simulink model "counter"  (R2021a)
settings: Solver=FixedStepDiscrete  StartTime=0.0  StopTime=10.0  RelTol=1e-3  EnableMultiTasking=on
settings Model: Creator=Noha  LastModifiedBy=Noha
settings DataIOCC: ReturnWorkspaceOutputs=off
settings OptimizationCC: DefaultParameterBehavior=Inlined  InlineInvariantSignals=on  EnableMemcpy=off  LifeSpan=1  EfficientTunableParamExpr=on
settings DebuggingCC: UnderspecifiedInitializationDetection=Classic  MergeDetectMultiDrivingBlocksExec=none  SFMachineParentedDataDiag=warning  ArithmeticOperatorsInVariantConditions=warning
settings ModelReferenceCC: PropagateSignalLabelsOutOfModel=off
settings SFSimCC: MATLABDynamicMemAlloc=off  CustomCodeUndefinedFunction=UseInterfaceOnly
settings RTWCC: SystemTargetFile=ert.tlc  GenCodeOnly=on  TemplateMakefile=ert_default_tmf  GenerateReport=on  IncludeHyperlinkInReport=on  LaunchReport=on  GenerateTraceInfo=on  GenerateTraceReport=on  GenerateTraceReportSl=on  GenerateTraceReportSf=on  GenerateTraceReportEml=on
settings CodeAppCC: ForceParamTrailComments=on  IgnoreCustomStorageClasses=off  OperatorAnnotations=on  SimulinkDataObjDesc=on  SFDataObjDesc=on  MATLABFcnDesc=on  InsertBlockDesc=on  StateflowObjectComments=on  MATLABSourceComments=on
settings ERTTargetCC: MultiwordLength=2048  GenerateSampleERTMain=on  InlinedParameterPlacement=NonHierarchical  ERTCustomFileTemplate=example_file_process.tlc

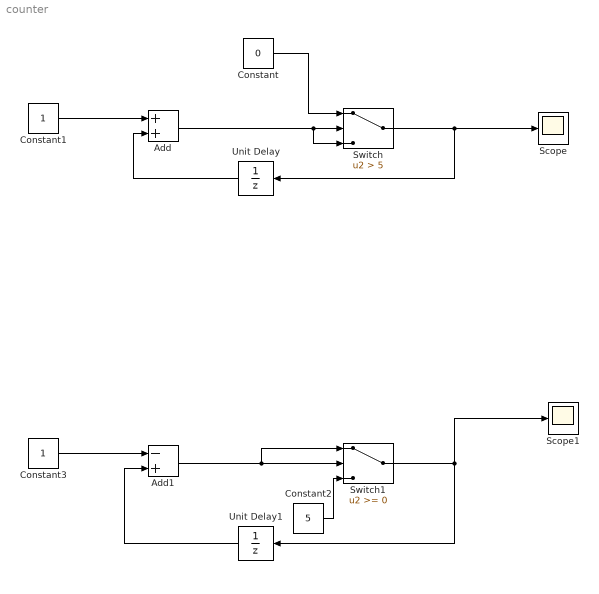
== system counter ==
  Add : Sum
  Add1 : Sum  Inputs=-+
  Constant : Constant  Value=0
  Constant1 : Constant
  Constant2 : Constant  Value=5
  Constant3 : Constant
  Scope : Scope
  Scope1 : Scope
  Switch : Switch  Criteria=u2 > Threshold  Threshold=5
  Switch1 : Switch
  Unit Delay : UnitDelay  SampleTime=-1  HasFrameUpgradeWarning=on
  Unit Delay1 : UnitDelay  InitialCondition=5  SampleTime=-1  HasFrameUpgradeWarning=on
  wires:
  Unit Delay/1 -> Add/2
  Add/1 -> Switch/3, Switch/2
  Switch/1 -> Unit Delay/1, Scope/1
  Constant/1 -> Switch/1
  Constant1/1 -> Add/1
  Constant3/1 -> Add1/1
  Switch1/1 -> Unit Delay1/1, Scope1/1
  Unit Delay1/1 -> Add1/2
  Constant2/1 -> Switch1/3
  Add1/1 -> Switch1/2, Switch1/1
